simulink model "inv_pend_three"  (R2022a)
settings: Solver=ode45  StartTime=0.0  StopTime=1  RelTol=1e-3  EnableMultiTasking=on
InitFcn:
  | clear functions
libraries: truetime x1
settings Model: ExtModeTrigMode=oneshot  ExtModeArmWhenConnect=off  Creator=anton  LastModifiedBy=pirmi
settings SolverCC: AlgebraicLoopSolver=TrustRegion
settings DataIOCC: SaveFormat=Array  SignalLoggingSaveFormat=ModelDataLogs  ReturnWorkspaceOutputs=off  OutputSaveName=Theta
settings OptimizationCC: BlockReduction=off  BooleanDataType=off  ExpressionDepthLimit=2147483647  LifeSpan=inf
settings DebuggingCC: SaveWithParameterizedLinksMsg=none  UnderspecifiedInitializationDetection=Classic  MergeDetectMultiDrivingBlocksExec=none  SignalResolutionControl=TryResolveAllWithWarning  MultiTaskDSMMsg=warning  MultiTaskCondExecSysMsg=none  FcnCallInpInsideContextMsg=warning  UnconnectedInputMsg=warning  UnconnectedOutputMsg=warning  UnconnectedLineMsg=warning  StateNameClashWarn=warning  SFUnexpectedBacktrackingDiag=warning  SFNoUnconditionalDefaultTransitionDiag=warning  SFExecutionAtInitializationDiag=none  SFMachineParentedDataDiag=warning  ArithmeticOperatorsInVariantConditions=warning
settings HardwareCC: ProdBitPerPointer=32  ProdBitPerSizeT=32  ProdBitPerPtrDiffT=32  ProdLargestAtomicFloat=None  ProdIntDivRoundTo=Undefined  ProdEndianess=Unspecified  ProdWordSize=32  ProdHWDeviceType=32-bit Generic  TargetUnknown=on
settings ModelReferenceCC: PropagateSignalLabelsOutOfModel=off
settings SFSimCC: SimUseLocalCustomCode=off  CustomCodeUndefinedFunction=UseInterfaceOnly
settings RTWCC: RTWUseLocalCustomCode=off
settings CodeAppCC: StateflowObjectComments=on
settings GRTTargetCC: TargetLangStandard=C89/C90 (ANSI)  CombineOutputUpdateFcns=off  GRTInterface=on
settings ConfigComp: CovMetricSettings=dw  CovSaveCumulativeToWorkspaceVar=on  CovSaveSingleToWorkspaceVar=on  CovExternalEMLEnable=off

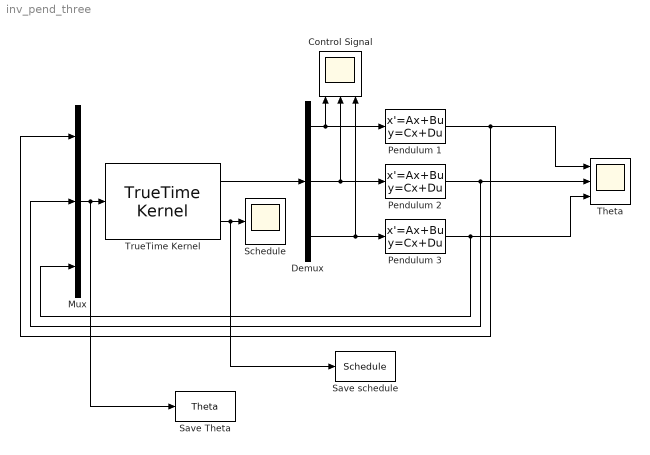
== system inv_pend_three ==
  Control Signal : Scope  NumInputPorts=3
  Demux : Demux  Outputs=3
      settings: DisplayOption=none
  Mux : Mux  Inputs=3
  Pendulum 1 : StateSpace  A=[0 3.0628;32 0]  B=[2; 0]  C=[0 1.5314]  D=0  InitialCondition=[0; 0.1]
  Pendulum 2 : StateSpace  A=[0 3.0625;16 0]  B=[2; 0]  C=[0 1.5313]  D=0  InitialCondition=[0; 0.10000]  AbsoluteTolerance=1e-6
  Pendulum 3 : StateSpace  A=[0 2.0306;16 0]  B=[2; 0]  C=[0 1.0153]  D=0  InitialCondition=[0;0.1]
  Save Theta : ToWorkspace  VariableName=Theta  SaveFormat=Structure With Time  SampleTime=-1
  Save schedule : ToWorkspace  VariableName=Schedule  SaveFormat=Structure  SampleTime=-1
  Schedule : Scope
  Theta : Scope  NumInputPorts=3
  TrueTime Kernel : truetime/TrueTime Kernel  sfun=init_pend_three  args=1  ninputsoutputs=[3 3]  ntriggers=0  trigtype=falling  nwnodenbr=[]  clockoffsetdrift=[0 0]  schedoutput=on  battery=off  poweroutput=off
  wires:
  Demux/2 -> Control Signal/2, Pendulum 2/1
  Demux/3 -> Control Signal/3, Pendulum 3/1
  Pendulum 1/1 -> Mux/1, Theta/1
  Pendulum 2/1 -> Mux/2, Theta/2
  Pendulum 3/1 -> Mux/3, Theta/3
  Mux/1 -> TrueTime Kernel/1, Save Theta/1
  TrueTime Kernel/1 -> Demux/1
  Demux/1 -> Control Signal/1, Pendulum 1/1
  TrueTime Kernel/2 -> Schedule/1, Save schedule/1
